simulink model "ex2"  (R2025b)
settings: Solver=VariableStepAuto  StartTime=0.0  StopTime=10.0  RelTol=1e-3
settings Model: Creator=vladl  LastModifiedBy=vladl

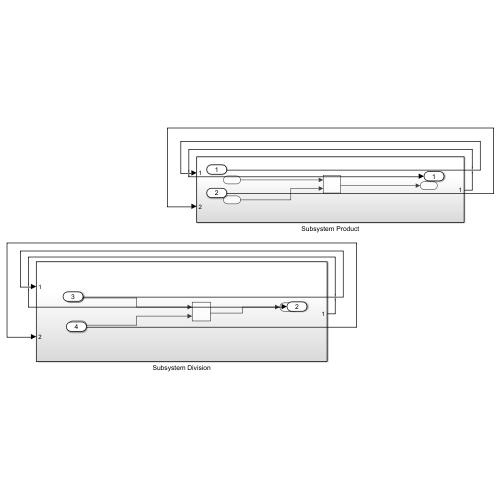
[thumbnail: Simulink's stored preview of the top-level diagram]
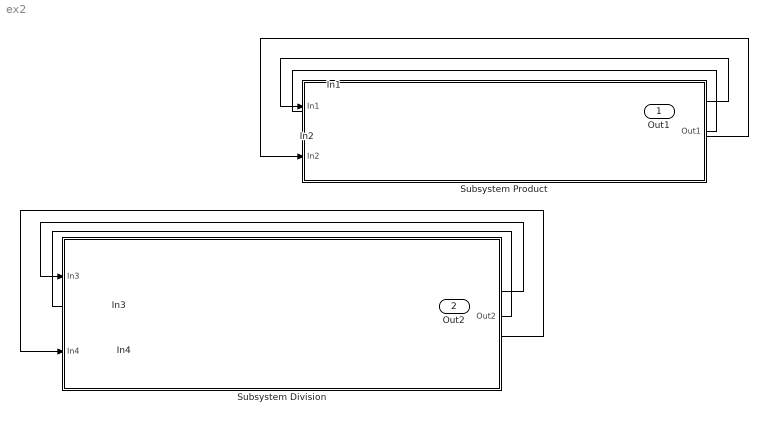
== system ex2 ==
  In1 : Inport
  In2 : Inport  Port=2
  In3 : Inport  Port=3
  In4 : Inport  Port=4
  Subsystem Division : Subsystem
  Subsystem Product : Subsystem
  Out1 : Outport
  Out2 : Outport  Port=2
  wires:
  In1/1 -> Subsystem Product/1(In1)
  In2/1 -> Subsystem Product/2(In2)
  Subsystem Product/1(Out1) -> Out1/1
  In3/1 -> Subsystem Division/1(In3)
  In4/1 -> Subsystem Division/2(In4)
  Subsystem Division/1(Out2) -> Out2/1

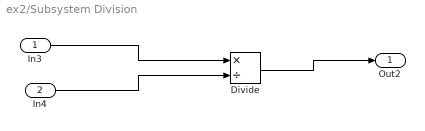
== system ex2/Subsystem Division ==
  In3 : Inport
  In4 : Inport  Port=2
  Divide : Product  Inputs=*/
  Out2 : Outport
  wires:
  In3/1 -> Divide/1
  In4/1 -> Divide/2
  Divide/1 -> Out2/1

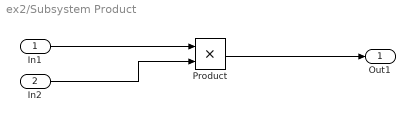
== system ex2/Subsystem Product ==
  In1 : Inport
  In2 : Inport  Port=2
  Product : Product
  Out1 : Outport
  wires:
  Product/1 -> Out1/1
  In1/1 -> Product/1
  In2/1 -> Product/2
